simulink model "CF012A_GmStrtStop"  (R2013b)
settings: Solver=FixedStepDiscrete  SolverMode=SingleTasking  StartTime=0.0  StopTime=1  FixedStep=0.002  RelTol=1e-3
values from neighbouring files (symbols this model uses):
  CNV100MICROSECTOMILLISEC_MILLISECPERCNT_F32 = DataDict.Constant    [CF012A_GmStrtStop_DataDict.m]
  DISMOD_CNT_U08 = DataDict.Constant    [CF012A_GmStrtStop_DataDict.m]
  DISMODRATE_ULSPERSEC_F32 = DataDict.Constant    [CF012A_GmStrtStop_DataDict.m]
  FLTMOD_CNT_U08 = DataDict.Constant    [CF012A_GmStrtStop_DataDict.m]
  GmStrtStopEna = DataDict.Calibration    [CF012A_GmStrtStop_DataDict.m]
  GmStrtStopFltRateLim = DataDict.Calibration    [CF012A_GmStrtStop_DataDict.m]
  GmStrtStopMod1ToStopRateLim = DataDict.Calibration    [CF012A_GmStrtStop_DataDict.m]
  GmStrtStopNormRateLim = DataDict.Calibration    [CF012A_GmStrtStop_DataDict.m]
  GmStrtStopNormToMod1RateLim = DataDict.Calibration    [CF012A_GmStrtStop_DataDict.m]
  GmStrtStopStopAndMod2RateLim = DataDict.Calibration    [CF012A_GmStrtStop_DataDict.m]
  GmStrtStopStopMod1Tmr = DataDict.Calibration    [CF012A_GmStrtStop_DataDict.m]
  GmStrtStopStopMod2Tmr = DataDict.Calibration    [CF012A_GmStrtStop_DataDict.m]
  MOD1_CNT_U08 = DataDict.Constant    [CF012A_GmStrtStop_DataDict.m]
  MOD2_CNT_U08 = DataDict.Constant    [CF012A_GmStrtStop_DataDict.m]
  NORMMOD_CNT_U08 = DataDict.Constant    [CF012A_GmStrtStop_DataDict.m]
  STOPMOD_CNT_U08 = DataDict.Constant    [CF012A_GmStrtStop_DataDict.m]
  STRTSTOPRATEHILIM_ULSPERSEC_F32 = DataDict.Constant    [CF012A_GmStrtStop_DataDict.m]
  STRTSTOPRATELOWRLIM_ULSPERSEC_F32 = DataDict.Constant    [CF012A_GmStrtStop_DataDict.m]
  STRTSTOPSCAHILIM_ULS_F32 = DataDict.Constant    [CF012A_GmStrtStop_DataDict.m]
  STRTSTOPSCALOWRLIM_ULS_F32 = DataDict.Constant    [CF012A_GmStrtStop_DataDict.m]
undefined symbols (not defined in the file or in its folder): u2, u3, u4, u5
libraries: FixdToFloat x2, NxtrLim x2, simulink x2
(part 1 of 4)
settings Model: Creator=rzp7hw  LastModifiedBy=sz7vy6
settings SolverCC: AutoInsertRateTranBlk=on  InsertRTBMode=Always
settings DataIOCC: LimitDataPoints=off  SaveFormat=Structure  ReturnWorkspaceOutputs=on
settings OptimizationCC: BlockReduction=off  InlineParams=on  ZeroExternalMemoryAtStartup=off  ZeroInternalMemoryAtStartup=off  OptimizeModelRefInitCode=on  LifeSpan=1
settings DebuggingCC: SignalInfNanChecking=error  SignalRangeChecking=warning  UnderspecifiedInitializationDetection=Simplified  SolverPrmCheckMsg=error  InheritedTsInSrcMsg=error  DiscreteInheritContinuousMsg=error  SingleTaskRateTransMsg=error  TasksWithSamePriorityMsg=error  SigSpecEnsureSampleTimeMsg=error  CheckMatrixSingularityMsg=error  ParameterUnderflowMsg=error  ParameterPrecisionLossMsg=error  ParameterTunabilityLossMsg=error  FixptConstUnderflowMsg=warning  FixptConstOverflowMsg=warning  VectorMatrixConversionMsg=error  SignalLabelMismatchMsg=error  UnconnectedInputMsg=error  UnconnectedOutputMsg=error  UnconnectedLineMsg=error  SFcnCompatibilityMsg=error  UniqueDataStoreMsg=warning  BusObjectLabelMismatch=error  RootOutportRequireBusObject=error  AssertControl=DisableAll  ModelReferenceIOMsg=error  ModelReferenceVersionMismatchMessage=warning  ModelReferenceIOMismatchMessage=error  ModelReferenceCSMismatchMessage=warning  ModelReferenceDataLoggingMessage=error  StateNameClashWarn=warning  StrictBusMsg=ErrorOnBusTreatedAsVector  NonBusSignalsTreatedAsBus=error  SFUnexpectedBacktrackingDiag=error  SFInvalidInputDataAccessInChartInitDiag=error  SFNoUnconditionalDefaultTransitionDiag=error  SFTransitionOutsideNaturalParentDiag=error  SFUnconditionalTransitionShadowingDiag=error  SFUndirectedBroadcastEventsDiag=error
settings ModelReferenceCC: ModelReferenceNumInstancesAllowed=Single
settings RTWCC: SystemTargetFile=autosar.tlc  GenCodeOnly=on  TemplateMakefile=ert_default_tmf  Description=AUTOSAR  GenerateReport=on  ProcessScript=autosar_make_rtw_hook  LaunchReport=on
settings CodeAppCC: GenerateComments=off  IgnoreCustomStorageClasses=off  CustomSymbolStrType=$N$R$M  CustomSymbolStrBlkIO=$N$M  SimulinkBlockComments=off
settings STFCustomTargetCC: ParMdlRefBuildCompliant=on  CompOptLevelCompliant=on  IncludeMdlTerminateFcn=off  CombineOutputUpdateFcns=on  SuppressErrorStatus=on  ERTFirstTimeCompliant=on  ERTCustomFileBanners=on  SupportNonFinite=off  SupportComplex=off  SupportContinuousTime=off  SupportNonInlinedSFcns=off  MATLABClassNameForMDSCustomization=Simulink.SoftwareTarget.ERTCustomization  AutosarCompliant=on  GRTInterface=off  SystemTargetFile=autosar.tlc
settings ERTTargetCC: CodeReplacementLibrary=ANSI_C  ConcurrentExecutionCompliant=off  IncludeMdlTerminateFcn=off  SuppressErrorStatus=on  SupportNonFinite=off  SupportComplex=off  ModelStepFunctionPrototypeControlCompliant=off  CPPClassGenCompliant=off  AutosarCompliant=on  InlinedParameterPlacement=NonHierarchical  ERTCustomFileTemplate=example_file_process.tlc  EnableUserReplacementTypes=on

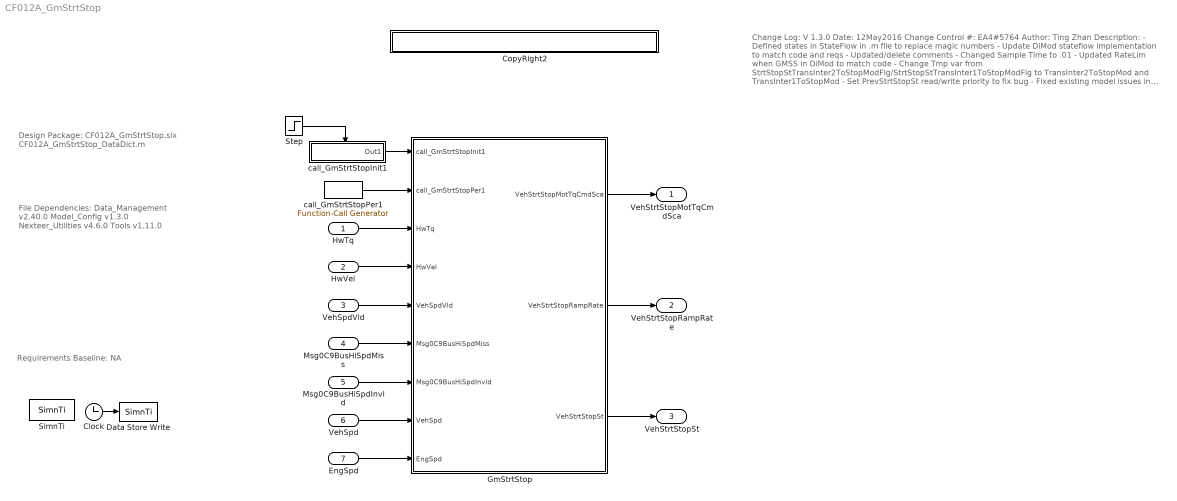
== system CF012A_GmStrtStop ==
  note: File Dependencies:
      |
      | Data_Management v2.40.0
      | Model_Config v1.3.0
      | Nexteer_Utilities v4.6.0
      | Tools v1.11.0
  note: Requirements Baseline: NA
  note: Change Log:
      |
      | V 1.3.0
      | Date: 12May2016
      | Change Control #: EA4#5764
      | Author: Ting Zhan
      |
      | Description:
      | - Defined states in StateFlow in .m file to replace magic numbers
      | - Update DiMod stateflow implementation to match code and reqs
      | - Updated/delete comments
      | - Changed Sample Time to .01
      | - Updated RateLim when GMSS in DiMod to match code
      | - Change Tmp var from StrtStopStTransInter2ToStopModFlg/StrtStopStTransInter1ToStopModFlg
      |  to TransInter2ToStopMod and TransInter1ToStopMod
      | - Set PrevStrtStopSt read/write priority to fix bug
      | - Fixed existing model issues in order to make model run
      |
      | V 1.2.0
      | Date: 08Feb2015
      | Change Control #: EA4#3589
      | Author: Sneha P (KPIT)
      | Description:
      |
      | - Replaced constant “MILLISECTO100MICROSECCNVN_CNT_F32” with
      |  “CNV100MICROSECTOMILLISEC_MILLISECPERCNT_F32“ in .m file
      | - Removed Millisec to 100Microsec coversion logic and implemented
      |   100Microsec(Cnt) to MilliSec conversion logic in model
      | Path:(CF012A_GmStrtStop/GmStrtStop/GmStrtStopPer1/StrtStopSt_Inter2ToStopModFlg/Elpse Ti)
      | and : (CF012A_GmStrtStop/GmStrtStop/GmStrtStopPer1/StrtStopSt_Inter1ToStopModFlg/Elpse Ti)
      | - Changed DocUnit of "GmStrtStopStopMod2Tmr" to "MilliSec" with
      |    respective change in Init, Min, Max values
      |
      |
      | V 1.1.0
      | Date: 29Jan2015
      | Change Control #: EA4#3589
      | Author: Sneha P (KPIT)
      | Description:
      |
      | - Changed maximum range of PIM variables 'PrevStrtStopSt' & 'PrevActSt'
      |   from 4 to 5 as per anomaly EA4#2621
      |
      | - Changed Init value of output signal 'StrtStopSca' from 0 to 1 as per
      |   anomaly CR EA4#3036
      |
      | - Following changes done as per anomaly CR#1886
      |
      |   - In .m file, calibration 'GmStrtStopStopMod1Tmr' changed to 'float32'
      |   - In .m file, PIMS 'Mod1RefTmr' and 'Mod2RefTmr' changed to 'uint32'
      |   - Constant 'TISTEP_MILLISEC_F32' to be removed from .m file.
      |   - Logic related to elapsed timers in state implemented in model
      |
      | - Data type of PIM variables 'Mod1RefTmr' and 'Mod2RefTmr' changed to uint32
      |   as per anomaly CR EA4#2991
      |
      |
      | V 1.0.0
      | Date: 8Jul2015
      | Change Control #: EA4#
      | Author: Qi Wang
      | Description:
      | - Initial Release Based on EA3V 1.0.0
      | CR#1623
  note: Design Package:
      | CF012A_GmStrtStop.slx
      | CF012A_GmStrtStop_DataDict.m
  HwTq : Inport  RequirementInfo={} %GIDa_a4d85b5d_ed9b_4901_a351_104e8322e8d5
  HwVel : Inport  RequirementInfo={} %GIDa_ecdde577_07ed_48f6_83d9_055f4ed5439e  Port=2
  VehSpdVld : Inport  Port=3
  Msg0C9BusHiSpdMiss : Inport  Port=4
  Msg0C9BusHiSpdInvld : Inport  Port=5
  VehSpd : Inport  RequirementInfo={} %GIDa_7789dff7_ea50_483a_835d_9871b9cb485d  Port=6
  EngSpd : Inport  RequirementInfo={} %GIDa_55b73ebd_28f3_4154_b330_73735b6396df  Port=7
  Clock : Clock
  CopyRight2 : Subsystem  Description=|  mask(Copyright Information){none=on}
      | Copyright info block.                                               
      |                                                                     
      | Place copyright information at the top of every subsystem in design.
      mask prompts: none "No parameters"
      mask help: Place copyright information at the top of every subsystem in design.
      mask Display:
      | NxtrConf = 'Nexteer Confidential';
      | 
      | sys = bdroot; %handle for the current model ("system")
      | first = get_param(sys,'Created');
      | if(isempty(first))
      |     first = datestr(now,'yyyy');
      | else
      |     first = first(end-3:end);  %year is last four digits
      | end
      | 
      | last = get_param(sys,'LastModifiedDate');
      | if isempty(last)
      |     last = datestr(now,'yyyy');
      | else
      |     last = last(end-3:end);
      | end
      | 
      | if strcmp(first,last)
      |     fprintf('%s -- Copyright %s Nexteer',NxtrConf,first)
      | else
      |     fprintf('%s -- %s%s- %s Nexteer',NxtrConf,char(169),first,last)
      | end
  Data Store Write : DataStoreWrite  DataStoreName=SimnTi
  GmStrtStop : Subsystem  RequirementInfo={} %GIDa_2223a9a7_07d3_48cf_9066_a6e132ab91db
  SimnTi : DataStoreMemory  DataStoreName=SimnTi
  Step : Step  Time=.002  Before=1  After=0  SampleTime=0
  call_GmStrtStopInit1 : Subsystem  TreatAsAtomicUnit=on
  call_GmStrtStopPer1 : simulink/Ports & Subsystems/Function-Call Generator  RequirementInfo={} %GIDa_054eadac_8b4f_4392_b7a2_0fbd071b25ae  sample_time=.01  numberOfIterations=1
      settings: AttributesFormatString=%<sample_time>
  VehStrtStopMotTqCmdSca : Outport  RequirementInfo={} %GIDa_bfe28696_5cd6_4f13_a500_f4d97106e76f
  VehStrtStopRampRate : Outport  RequirementInfo={} %GIDa_064db67c_6e20_4c88_b4e7_4e0dfc6b8609  Port=2
  VehStrtStopSt : Outport  RequirementInfo={} %GIDa_5adf65af_5735_4113_a387_e1ee48936d3d  Port=3
  wires:
  call_GmStrtStopPer1/1 -> GmStrtStop/2(call_GmStrtStopPer1)
  HwTq/1 -> GmStrtStop/3(HwTq)
  HwVel/1 -> GmStrtStop/4(HwVel)
  VehSpdVld/1 -> GmStrtStop/5(VehSpdVld)
  Msg0C9BusHiSpdMiss/1 -> GmStrtStop/6(Msg0C9BusHiSpdMiss)
  Msg0C9BusHiSpdInvld/1 -> GmStrtStop/7(Msg0C9BusHiSpdInvld)
  VehSpd/1 -> GmStrtStop/8(VehSpd)
  EngSpd/1 -> GmStrtStop/9(EngSpd)
  GmStrtStop/1(VehStrtStopMotTqCmdSca) -> VehStrtStopMotTqCmdSca/1
  GmStrtStop/2(VehStrtStopRampRate) -> VehStrtStopRampRate/1
  GmStrtStop/3(VehStrtStopSt) -> VehStrtStopSt/1
  Step/1 -> call_GmStrtStopInit1/Enable
  call_GmStrtStopInit1/1(Out1) -> GmStrtStop/1(call_GmStrtStopInit1)
  Clock/1 -> Data Store Write/1

== system CF012A_GmStrtStop/CopyRight2 ==

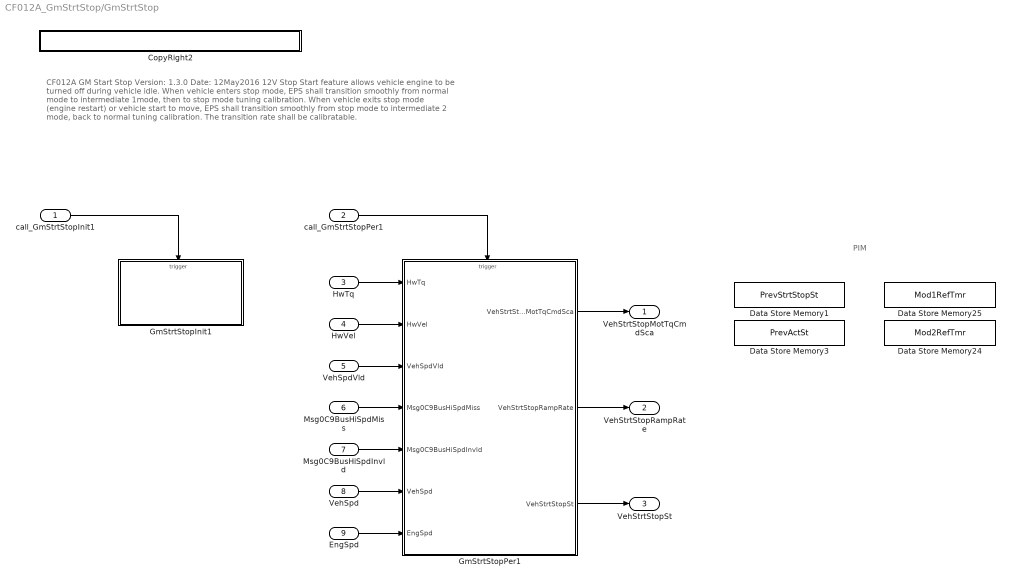
== system CF012A_GmStrtStop/GmStrtStop ==
  note: PIM
  note: CF012A GM Start Stop
      | Version: 1.3.0      Date: 12May2016
      |
      | 12V Stop Start feature allows vehicle engine to be turned off during vehicle idle. When vehicle enters stop mode, EPS shall transition smoothly from
      | normal mode to intermediate 1mode, then to stop mode tuning calibration.  When vehicle exits stop mode (engine restart) or vehicle start to move, EPS shall
      | transition smoothly from stop mode to intermediate 2 mode, back to normal tuning calibration.  The transition rate shall be calibratable.
  call_GmStrtStopInit1 : Inport  RequirementInfo={} %GIDa_e66133ce_4d9a_4583_9cdf_9b3fe85f0c43
  call_GmStrtStopPer1 : Inport  RequirementInfo={} %GIDa_29356ae4_ffe9_446f_a246_ff587b699871  Port=2
  HwTq : Inport  RequirementInfo="{'linktype_rmi_doors' '0000c6e0 (/GM T1XX/SubSystem Specifications/Customer Functions/CF012 12V Start Stop)' '#9' 'true' 'REQ:  9' '' } %GIDa_b59c9030_1f31_468f_8592_3e6a0470c9b8"  Port=3
  HwVel : Inport  RequirementInfo="{'linktype_rmi_doors' '0000c6e0 (/GM T1XX/SubSystem Specifications/Customer Functions/CF012 12V Start Stop)' '#32' 'true' 'REQ:  32' '' } %GIDa_d97376d2_3983_4ccc_a2b9_13e32f4f2e19"  Port=4
  VehSpdVld : Inport  RequirementInfo="{'linktype_rmi_doors' '0000c6e0 (/GM T1XX/SubSystem Specifications/Customer Functions/CF012 12V Start Stop)' '#33' 'true' 'REQ:  33' '' } %GIDa_855152bf_675c_4d82_87df_76d2e9253c11"  Port=5
  Msg0C9BusHiSpdMiss : Inport  RequirementInfo="{'linktype_rmi_doors' '0000c6e0 (/GM T1XX/SubSystem Specifications/Customer Functions/CF012 12V Start Stop)' '#73' 'true' 'REQ:  73' '' } %GIDa_4764eb12_da95_4964_a18b_bc9ea30562ea"  Port=6
  Msg0C9BusHiSpdInvld : Inport  RequirementInfo="{'linktype_rmi_doors' '0000c6e0 (/GM T1XX/SubSystem Specifications/Customer Functions/CF012 12V Start Stop)' '#221' 'true' 'REQ:  221' '' } %GIDa_0435394c_4b65_4e7a_927b_eb164670af9f"  Port=7
  VehSpd : Inport  RequirementInfo="{'linktype_rmi_doors' '0000c6e0 (/GM T1XX/SubSystem Specifications/Customer Functions/CF012 12V Start Stop)' '#36' 'true' 'REQ:  36' '' } %GIDa_26fe1dc3_440c_4c24_809e_674d3c570084"  Port=8
  EngSpd : Inport  RequirementInfo="{'linktype_rmi_doors' '0000c6e0 (/GM T1XX/SubSystem Specifications/Customer Functions/CF012 12V Start Stop)' '#37' 'true' 'REQ:  37' '' } %GIDa_1a15c7f1_c702_477b_b228_a391a493889d"  Port=9
  CopyRight2 : Subsystem  Description=|  mask(Copyright Information){none=on}
      | Copyright info block.                                               
      |                                                                     
      | Place copyright information at the top of every subsystem in design.
      mask prompts: none "No parameters"
      mask help: Place copyright information at the top of every subsystem in design.
      mask Display:
      | NxtrConf = 'Nexteer Confidential';
      | 
      | sys = bdroot; %handle for the current model ("system")
      | first = get_param(sys,'Created');
      | if(isempty(first))
      |     first = datestr(now,'yyyy');
      | else
      |     first = first(end-3:end);  %year is last four digits
      | end
      | 
      | last = get_param(sys,'LastModifiedDate');
      | if isempty(last)
      |     last = datestr(now,'yyyy');
      | else
      |     last = last(end-3:end);
      | end
      | 
      | if strcmp(first,last)
      |     fprintf('%s -- Copyright %s Nexteer',NxtrConf,first)
      | else
      |     fprintf('%s -- %s%s- %s Nexteer',NxtrConf,char(169),first,last)
      | end
  Data Store Memory1 : DataStoreMemory  DataStoreName=PrevStrtStopSt  StateMustResolveToSignalObject=on
  Data Store Memory24 : DataStoreMemory  DataStoreName=Mod2RefTmr  StateMustResolveToSignalObject=on
  Data Store Memory25 : DataStoreMemory  DataStoreName=Mod1RefTmr  StateMustResolveToSignalObject=on
  Data Store Memory3 : DataStoreMemory  DataStoreName=PrevActSt  StateMustResolveToSignalObject=on
  GmStrtStopInit1 : Subsystem
  GmStrtStopPer1 : Subsystem
  VehStrtStopMotTqCmdSca : Outport  RequirementInfo="{'linktype_rmi_doors' '0000c6e0 (/GM T1XX/SubSystem Specifications/Customer Functions/CF012 12V Start Stop)' '#11' 'true' 'REQ:  11' '' } %GIDa_548d980c_3c7b_491e_a0fa_0c64e6562fc0"
  VehStrtStopRampRate : Outport  RequirementInfo="{'linktype_rmi_doors' '0000c6e0 (/GM T1XX/SubSystem Specifications/Customer Functions/CF012 12V Start Stop)' '#40' 'true' 'REQ:  40' '' } %GIDa_43ddaf5d_aaf1_4964_b6d5_b32b85f57a27"  Port=2
  VehStrtStopSt : Outport  RequirementInfo="{'linktype_rmi_doors' '0000c6e0 (/GM T1XX/SubSystem Specifications/Customer Functions/CF012 12V Start Stop)' '#216' 'true' 'REQ:  216' '' } %GIDa_fd34a469_cf67_4bd9_a2b8_b0cdcd42aa93"  Port=3
  wires:
  HwTq/1 -> GmStrtStopPer1/1(HwTq)
  HwVel/1 -> GmStrtStopPer1/2(HwVel)
  VehSpd/1 -> GmStrtStopPer1/6(VehSpd)
  EngSpd/1 -> GmStrtStopPer1/7(EngSpd)
  GmStrtStopPer1/1(VehStrtStopMotTqCmdSca) -> VehStrtStopMotTqCmdSca/1
  GmStrtStopPer1/2(VehStrtStopRampRate) -> VehStrtStopRampRate/1
  call_GmStrtStopPer1/1 -> GmStrtStopPer1/Trigger
  GmStrtStopPer1/3(VehStrtStopSt) -> VehStrtStopSt/1
  Msg0C9BusHiSpdInvld/1 -> GmStrtStopPer1/5(Msg0C9BusHiSpdInvld)
  Msg0C9BusHiSpdMiss/1 -> GmStrtStopPer1/4(Msg0C9BusHiSpdMiss)
  VehSpdVld/1 -> GmStrtStopPer1/3(VehSpdVld)
  call_GmStrtStopInit1/1 -> GmStrtStopInit1/Trigger

== system CF012A_GmStrtStop/call_GmStrtStopInit1 ==
  Enable : EnablePort
  CopyRight2 : Subsystem  Description=|  mask(Copyright Information){none=on}
      | Copyright info block.                                               
      |                                                                     
      | Place copyright information at the top of every subsystem in design.
      mask prompts: none "No parameters"
      mask help: Place copyright information at the top of every subsystem in design.
      mask Display:
      | NxtrConf = 'Nexteer Confidential';
      | 
      | sys = bdroot; %handle for the current model ("system")
      | first = get_param(sys,'Created');
      | if(isempty(first))
      |     first = datestr(now,'yyyy');
      | else
      |     first = first(end-3:end);  %year is last four digits
      | end
      | 
      | last = get_param(sys,'LastModifiedDate');
      | if isempty(last)
      |     last = datestr(now,'yyyy');
      | else
      |     last = last(end-3:end);
      | end
      | 
      | if strcmp(first,last)
      |     fprintf('%s -- Copyright %s Nexteer',NxtrConf,first)
      | else
      |     fprintf('%s -- %s%s- %s Nexteer',NxtrConf,char(169),first,last)
      | end
  Function-Call Generator : simulink/Ports & Subsystems/Function-Call Generator  sample_time=.01  numberOfIterations=1
  Out1 : Outport
  wires:
  Function-Call Generator/1 -> Out1/1

== system CF012A_GmStrtStop/GmStrtStop/CopyRight2 ==

== system CF012A_GmStrtStop/GmStrtStop/GmStrtStopInit1 ==
  function : TriggerPort  TriggerType=function-call
  CopyRight2 : Subsystem  Description=|  mask(Copyright Information){none=on}
      | Copyright info block.                                               
      |                                                                     
      | Place copyright information at the top of every subsystem in design.
      mask prompts: none "No parameters"
      mask help: Place copyright information at the top of every subsystem in design.
      mask Display:
      | NxtrConf = 'Nexteer Confidential';
      | 
      | sys = bdroot; %handle for the current model ("system")
      | first = get_param(sys,'Created');
      | if(isempty(first))
      |     first = datestr(now,'yyyy');
      | else
      |     first = first(end-3:end);  %year is last four digits
      | end
      | 
      | last = get_param(sys,'LastModifiedDate');
      | if isempty(last)
      |     last = datestr(now,'yyyy');
      | else
      |     last = last(end-3:end);
      | end
      | 
      | if strcmp(first,last)
      |     fprintf('%s -- Copyright %s Nexteer',NxtrConf,first)
      | else
      |     fprintf('%s -- %s%s- %s Nexteer',NxtrConf,char(169),first,last)
      | end
  Data Store Write4 : DataStoreWrite  RequirementInfo="{'linktype_rmi_doors' '0000c6e0 (/GM T1XX/SubSystem Specifications/Customer Functions/CF012 12V Start Stop)' '#161' 'true' 'REQ:  161' '' } %GIDa_5ca1f0f5_5840_49db_9093_aa24770101e9"  DataStoreName=Mod2RefTmr
  Data Store Write5 : DataStoreWrite  RequirementInfo="{'linktype_rmi_doors' '0000c6e0 (/GM T1XX/SubSystem Specifications/Customer Functions/CF012 12V Start Stop)' '#149' 'true' 'REQ:  149' '' } %GIDa_d8f43907_f50d_4586_b279_7eacc1f075da"  DataStoreName=Mod1RefTmr
  GetRefTmr100MicroSec32bit : Subsystem  RequirementInfo="{'linktype_rmi_doors' '0000c6e0 (/GM T1XX/SubSystem Specifications/Customer Functions/CF012 12V Start Stop)' '#161' 'true' 'REQ:  161' '' ; 'linktype_rmi_doors' '0000c6e0 (/GM T1XX/SubSystem Specifications/Customer Functions/CF012 12V Start Stop)' '#149' 'true' 'REQ:  149' '' } %GIDa_033bf37f_1dc6_42f0_a9e6_3056b3737b66"
  wires:
  GetRefTmr100MicroSec32bit/1(RefTmr) -> Data Store Write4/1, Data Store Write5/1

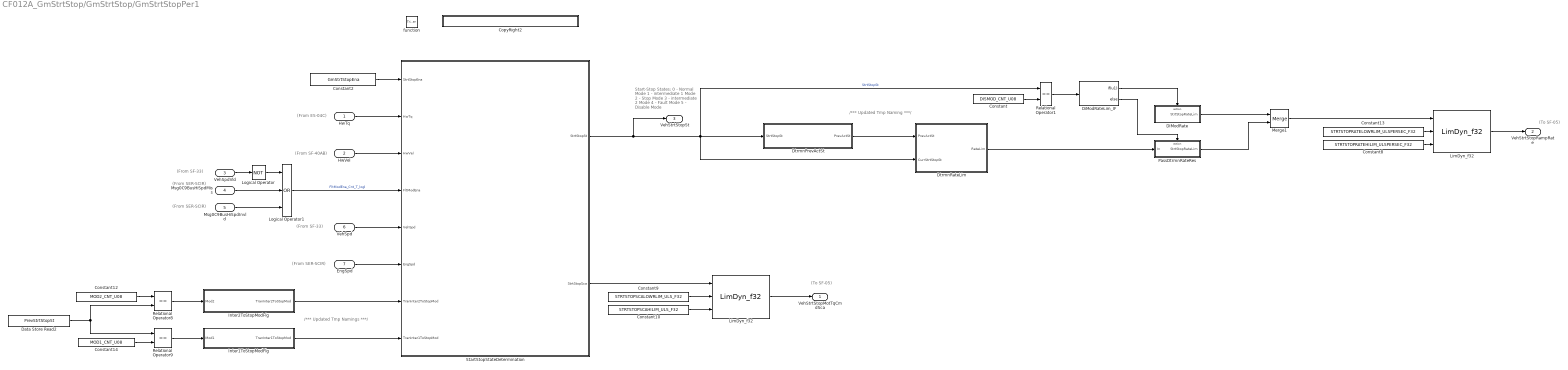
== system CF012A_GmStrtStop/GmStrtStop/GmStrtStopPer1 ==
  note: (From SER-SCIR)
  note: (From SF-33)
  note: (From SF-33)
  note: (From ES-04C)
  note: (From SF-40AB)
  note: Start-Stop States:
      |     0 - Normal Mode
      |     1 - intermediate 1 Mode
      |     2 - Stop Mode
      |     3 - intermediate 2 Mode
      |     4 - Fault Mode
      |     5 - Disable Mode
  note: (To SF-05)
  note: (To SF-05)
  note: (From SER-SCIR)
  note: (From SER-SCIR)
  note: /*** Updated Tmp Naming ***/
  note: /*** Updated Tmp Namings ***/
  HwTq : Inport  RequirementInfo="{'linktype_rmi_doors' '0000c6e0 (/GM T1XX/SubSystem Specifications/Customer Functions/CF012 12V Start Stop)' '#9' 'true' 'REQ:  9' '' } %GIDa_42b69aa0_42a4_4740_8c59_976a11e7f2ed"
  HwVel : Inport  RequirementInfo="{'linktype_rmi_doors' '0000c6e0 (/GM T1XX/SubSystem Specifications/Customer Functions/CF012 12V Start Stop)' '#32' 'true' 'REQ:  32' '' } %GIDa_ce32f278_8b5d_4046_b147_1f30eda0ac5e"  Port=2
  VehSpdVld : Inport  RequirementInfo="{'linktype_rmi_doors' '0000c6e0 (/GM T1XX/SubSystem Specifications/Customer Functions/CF012 12V Start Stop)' '#33' 'true' 'REQ:  33' '' } %GIDa_5065ff7a_d581_4098_bd8a_dd99a06fb2d8"  Port=3
  Msg0C9BusHiSpdMiss : Inport  RequirementInfo="{'linktype_rmi_doors' '0000c6e0 (/GM T1XX/SubSystem Specifications/Customer Functions/CF012 12V Start Stop)' '#73' 'true' 'REQ:  73' '' } %GIDa_81f8689f_bedf_48cc_9965_5d5e08e37da1"  Port=4
  Msg0C9BusHiSpdInvld : Inport  RequirementInfo="{'linktype_rmi_doors' '0000c6e0 (/GM T1XX/SubSystem Specifications/Customer Functions/CF012 12V Start Stop)' '#221' 'true' 'REQ:  221' '' } %GIDa_2c4353c3_7199_496f_b5e4_ca48d4fdc361"  Port=5
  VehSpd : Inport  RequirementInfo="{'linktype_rmi_doors' '0000c6e0 (/GM T1XX/SubSystem Specifications/Customer Functions/CF012 12V Start Stop)' '#36' 'true' 'REQ:  36' '' } %GIDa_778ed2e2_bf34_46d0_bd92_dde0215ed3d0"  Port=6
  EngSpd : Inport  RequirementInfo="{'linktype_rmi_doors' '0000c6e0 (/GM T1XX/SubSystem Specifications/Customer Functions/CF012 12V Start Stop)' '#37' 'true' 'REQ:  37' '' } %GIDa_ceeb79ba_05d2_485d_8198_e45df6d9a78c"  Port=7
  function : TriggerPort  TriggerType=function-call
  Constant : Constant  RequirementInfo="{'linktype_rmi_doors' '0000c6e0 (/GM T1XX/SubSystem Specifications/Customer Functions/CF012 12V Start Stop)' '#224' 'true' 'REQ:  224' '' } %GIDa_561b1e7e_3960_4a83_833c_80ef798b62ac"  Value=DISMOD_CNT_U08
  Constant10 : Constant  RequirementInfo="{'linktype_rmi_doors' '0000c6e0 (/GM T1XX/SubSystem Specifications/Customer Functions/CF012 12V Start Stop)' '#11' 'true' 'REQ:  11' '' } %GIDa_0c487a41_a1a4_450c_934d_c18e6ddbeebb"  Value=STRTSTOPSCAHILIM_ULS_F32
  Constant12 : Constant  RequirementInfo="{'linktype_rmi_doors' '0000c6e0 (/GM T1XX/SubSystem Specifications/Customer Functions/CF012 12V Start Stop)' '#161' 'true' 'REQ:  161' '' } %GIDa_bd66a335_3060_4277_b6ba_17e2ef32d7e1"  Value=MOD2_CNT_U08
  Constant13 : Constant  RequirementInfo="{'linktype_rmi_doors' '0000c6e0 (/GM T1XX/SubSystem Specifications/Customer Functions/CF012 12V Start Stop)' '#40' 'true' 'REQ:  40' '' } %GIDa_7a48ffb4_78e6_42f2_aec5_f8db377a48d6"  Value=STRTSTOPRATELOWRLIM_ULSPERSEC_F32
  Constant14 : Constant  RequirementInfo="{'linktype_rmi_doors' '0000c6e0 (/GM T1XX/SubSystem Specifications/Customer Functions/CF012 12V Start Stop)' '#149' 'true' 'REQ:  149' '' } %GIDa_d624ad54_41a1_4556_8a85_b9999226efec"  Value=MOD1_CNT_U08
  Constant2 : Constant  RequirementInfo="{'linktype_rmi_doors' '0000c6e0 (/GM T1XX/SubSystem Specifications/Customer Functions/CF012 12V Start Stop)' '#167' 'true' 'REQ:  167' '' ; 'linktype_rmi_doors' '0000c6e0 (/GM T1XX/SubSystem Specifications/Customer Functions/CF012 12V Start Stop)' '#225' 'true' 'REQ:  225' '' } %GIDa_4a6d5448_9282_48ab_99f6_9d1d9d9c576e"  Value=GmStrtStopEna  OutDataTypeStr=single
  Constant8 : Constant  RequirementInfo="{'linktype_rmi_doors' '0000c6e0 (/GM T1XX/SubSystem Specifications/Customer Functions/CF012 12V Start Stop)' '#40' 'true' 'REQ:  40' '' } %GIDa_a36f5600_300f_402a_9cfb_cda0992e5733"  Value=STRTSTOPRATEHILIM_ULSPERSEC_F32
  Constant9 : Constant  RequirementInfo="{'linktype_rmi_doors' '0000c6e0 (/GM T1XX/SubSystem Specifications/Customer Functions/CF012 12V Start Stop)' '#11' 'true' 'REQ:  11' '' } %GIDa_09a6d7e0_4b74_46ca_8329_69c0f542f506"  Value=STRTSTOPSCALOWRLIM_ULS_F32
  CopyRight2 : Subsystem  Description=|  mask(Copyright Information){none=on}
      | Copyright info block.                                               
      |                                                                     
      | Place copyright information at the top of every subsystem in design.
      mask prompts: none "No parameters"
      mask help: Place copyright information at the top of every subsystem in design.
      mask Display:
      | NxtrConf = 'Nexteer Confidential';
      | 
      | sys = bdroot; %handle for the current model ("system")
      | first = get_param(sys,'Created');
      | if(isempty(first))
      |     first = datestr(now,'yyyy');
      | else
      |     first = first(end-3:end);  %year is last four digits
      | end
      | 
      | last = get_param(sys,'LastModifiedDate');
      | if isempty(last)
      |     last = datestr(now,'yyyy');
      | else
      |     last = last(end-3:end);
      | end
      | 
      | if strcmp(first,last)
      |     fprintf('%s -- Copyright %s Nexteer',NxtrConf,first)
      | else
      |     fprintf('%s -- %s%s- %s Nexteer',NxtrConf,char(169),first,last)
      | end
  DIModRate : Subsystem  RequirementInfo="{'linktype_rmi_doors' '0000c6e0 (/GM T1XX/SubSystem Specifications/Customer Functions/CF012 12V Start Stop)' '#224' 'true' 'REQ:  224' '' } %GIDa_cf64ce6a_5fba_49e3_8042_142212826b91"  TreatAsAtomicUnit=on
  Data Store Read2 : DataStoreRead  RequirementInfo="{'linktype_rmi_doors' '0000c6e0 (/GM T1XX/SubSystem Specifications/Customer Functions/CF012 12V Start Stop)' '#149' 'true' 'REQ:  149' '' ; 'linktype_rmi_doors' '0000c6e0 (/GM T1XX/SubSystem Specifications/Customer Functions/CF012 12V Start Stop)' '#161' 'true' 'REQ:  161' '' } %GIDa_8d9c1ce9_7c89_423f_9be9_4e5c944f3999"  DataStoreName=PrevStrtStopSt
  DiModRateLim_IF : If  RequirementInfo="{'linktype_rmi_doors' '0000c6e0 (/GM T1XX/SubSystem Specifications/Customer Functions/CF012 12V Start Stop)' '#224' 'true' 'REQ:  224' '' } %GIDa_038e327d_895d_4c44_8a2d_683ea8b3fc41"  IfExpression=u1
  DtrmnPrevActSt : Subsystem  RequirementInfo="{'linktype_rmi_doors' '0000c6e0 (/GM T1XX/SubSystem Specifications/Customer Functions/CF012 12V Start Stop)' '#188' 'true' 'REQ:  188' '' } %GIDa_38faffb5_a6c9_485e_beed_5aff9cc6285a"
  DtrmnRateLim : Subsystem  RequirementInfo="{'linktype_rmi_doors' '0000c6e0 (/GM T1XX/SubSystem Specifications/Customer Functions/CF012 12V Start Stop)' '#86' 'true' 'REQ:  86' '' ; 'linktype_rmi_doors' '0000c6e0 (/GM T1XX/SubSystem Specifications/Customer Functions/CF012 12V Start Stop)' '#86' 'true' 'REQ:  86' '' ; 'linktype_rmi_doors' '0000c6e0 (/GM T1XX/SubSystem Specifications/Customer Functions/CF012 12V Start Stop)' '#86' 'true' 'REQ:  86' '' ; 'linktype_rmi_doors' '0000c6e0 (/GM T1XX/SubSystem Specifications/Customer Functions/CF012 12V Start Stop)' '#86' 'true' 'REQ:  86' '' ; 'linktype_rmi_doors' '0000c6e0 (/GM T1XX/SubSystem Specifications/Customer Functions/CF012 12V Start Stop)' '#86' 'true' 'REQ:  86' '' ; 'linktype_rmi_doors' '0000c6e0 (/GM T1XX/SubSystem Specifications/Customer Functions/CF012 12V Start Stop)' '#86' 'true' 'REQ:  86' '' ; 'linktype_rmi_doors' '0000c6e0 (/GM T1XX/SubSystem Specifications/Customer Functions/CF012 12V Start Stop)' '#86' 'true' 'REQ:  86' '' ; 'linktype_rmi_doors' '0000c6e0 (/GM T1XX/SubSystem Specifications/Customer Functions/CF012 12V Start Stop)' '#86' 'true' 'REQ:  86' '' } %GIDa_299b1b09_a509_4cb4_84f5_ba180b901640"
  Inter1ToStopModFlg : Subsystem  RequirementInfo="{'linktype_rmi_doors' '0000c6e0 (/GM T1XX/SubSystem Specifications/Customer Functions/CF012 12V Start Stop)' '#149' 'true' 'REQ:  149' '' } %GIDa_f6a3c2ac_6653_4871_9b62_0dad353837e0"
  Inter2ToStopModFlg : Subsystem  RequirementInfo="{'linktype_rmi_doors' '0000c6e0 (/GM T1XX/SubSystem Specifications/Customer Functions/CF012 12V Start Stop)' '#161' 'true' 'REQ:  161' '' } %GIDa_237f332d_7f17_42d1_8ac2_b1f2b09eedb1"
  LimDyn_f32 : NxtrLim/LimDyn_f32  RequirementInfo="{'linktype_rmi_doors' '0000c6e0 (/GM T1XX/SubSystem Specifications/Customer Functions/CF012 12V Start Stop)' '#40' 'true' 'REQ:  40' '' } %GIDa_8dd4f5c4_8b44_41f4_a726_2d8ed3933d71"
  "LimDyn_f32 " : NxtrLim/LimDyn_f32  RequirementInfo="{'linktype_rmi_doors' '0000c6e0 (/GM T1XX/SubSystem Specifications/Customer Functions/CF012 12V Start Stop)' '#11' 'true' 'REQ:  11' '' } %GIDa_7f5cde65_aec4_4b2d_989f_08b7e75f57e7"
  Logical Operator : Logic  RequirementInfo="{'linktype_rmi_doors' '0000c6e0 (/GM T1XX/SubSystem Specifications/Customer Functions/CF012 12V Start Stop)' '#62' 'true' 'REQ:  62' '' } %GIDa_656b04b2_cd99_48f1_ac88_88cf48a7ecb0"  Operator=NOT  AllPortsSameDT=off  OutDataTypeStr=boolean
  Logical Operator1 : Logic  RequirementInfo="{'linktype_rmi_doors' '0000c6e0 (/GM T1XX/SubSystem Specifications/Customer Functions/CF012 12V Start Stop)' '#62' 'true' 'REQ:  62' '' } %GIDa_76727bc4_1e34_4aba_9373_5b27799bfd27"  Operator=OR  Inputs=3  AllPortsSameDT=off  OutDataTypeStr=boolean
  Merge1 : Merge  RequirementInfo="{'linktype_rmi_doors' '0000c6e0 (/GM T1XX/SubSystem Specifications/Customer Functions/CF012 12V Start Stop)' '#224' 'true' 'REQ:  224' '' } %GIDa_d024fa85_1cfa_401c_a369_23d7beb805e7"
  PassDtrmnRateRes : Subsystem  RequirementInfo="{'linktype_rmi_doors' '0000c6e0 (/GM T1XX/SubSystem Specifications/Customer Functions/CF012 12V Start Stop)' '#224' 'true' 'REQ:  224' '' } %GIDa_3f3bc633_468d_4c4a_b40c_e9cb87a46491"  TreatAsAtomicUnit=on
  Relational Operator1 : RelationalOperator  RequirementInfo="{'linktype_rmi_doors' '0000c6e0 (/GM T1XX/SubSystem Specifications/Customer Functions/CF012 12V Start Stop)' '#224' 'true' 'REQ:  224' '' } %GIDa_4e8ea01d_c3d6_4af6_979b_c7f1ad0648af"  Operator===  OutDataTypeStr=boolean
  Relational Operator8 : RelationalOperator  RequirementInfo="{'linktype_rmi_doors' '0000c6e0 (/GM T1XX/SubSystem Specifications/Customer Functions/CF012 12V Start Stop)' '#161' 'true' 'REQ:  161' '' } %GIDa_33121b5f_7920_406b_86ac_c7c8173ab72f"  Operator===  OutDataTypeStr=boolean
  Relational Operator9 : RelationalOperator  RequirementInfo="{'linktype_rmi_doors' '0000c6e0 (/GM T1XX/SubSystem Specifications/Customer Functions/CF012 12V Start Stop)' '#149' 'true' 'REQ:  149' '' } %GIDa_4c13c417_adfb_409e_9fd6_df832113dce8"  Operator===  OutDataTypeStr=boolean
  StartStopStateDetermination : Stateflow chart  RequirementInfo="{'linktype_rmi_doors' '0000c6e0 (/GM T1XX/SubSystem Specifications/Customer Functions/CF012 12V Start Stop)' '#86' 'true' 'REQ:  86' '' ; 'linktype_rmi_doors' '0000c6e0 (/GM T1XX/SubSystem Specifications/Customer Functions/CF012 12V Start Stop)' '#166' 'true' 'REQ:  166' '' } %GIDa_c43b243b_0ee6_40fb_9826_be8530fa02b0"  TreatAsAtomicUnit=on  VariantControl=Variant1
  VehStrtStopMotTqCmdSca : Outport  RequirementInfo="{'linktype_rmi_doors' '0000c6e0 (/GM T1XX/SubSystem Specifications/Customer Functions/CF012 12V Start Stop)' '#11' 'true' 'REQ:  11' '' } %GIDa_cf5c80f6_4e22_46d3_8a7e_cf1a6ce51e5a"
  VehStrtStopRampRate : Outport  RequirementInfo="{'linktype_rmi_doors' '0000c6e0 (/GM T1XX/SubSystem Specifications/Customer Functions/CF012 12V Start Stop)' '#40' 'true' 'REQ:  40' '' } %GIDa_bd18f9ff_e11a_445b_ba9a_868b7e7cdcb3"  Port=2
  VehStrtStopSt : Outport  RequirementInfo="{'linktype_rmi_doors' '0000c6e0 (/GM T1XX/SubSystem Specifications/Customer Functions/CF012 12V Start Stop)' '#216' 'true' 'REQ:  216' '' } %GIDa_3f167dff_2f2a_4c61_8d63_f420465aae9f"  Port=3
  wires:
  HwVel/1 -> StartStopStateDetermination/3(HwVel)
  Logical Operator1/1 -> StartStopStateDetermination/4(FltModEna)  "FltModEna_Cnt_T_logl"
  EngSpd/1 -> StartStopStateDetermination/6(EngSpd)
  VehSpd/1 -> StartStopStateDetermination/5(VehSpd)
  HwTq/1 -> StartStopStateDetermination/2(HwTq)
  Constant2/1 -> StartStopStateDetermination/1(StrtStopEna)
  "LimDyn_f32 "/1 -> VehStrtStopMotTqCmdSca/1
  VehSpdVld/1 -> Logical Operator/1
  Logical Operator/1 -> Logical Operator1/1
  Msg0C9BusHiSpdMiss/1 -> Logical Operator1/2
  Msg0C9BusHiSpdInvld/1 -> Logical Operator1/3
  Constant/1 -> Relational Operator1/2
  Relational Operator1/1 -> DiModRateLim_IF/1
  DiModRateLim_IF/1 -> DIModRate/Action
  DiModRateLim_IF/2 -> PassDtrmnRateRes/Action
  PassDtrmnRateRes/1(StrtStopRateLim) -> Merge1/2
  DIModRate/1(StrtStopRateLim) -> Merge1/1
  StartStopStateDetermination/1(StrtStopSt) -> Relational Operator1/1, DtrmnPrevActSt/1(StrtStopSt), DtrmnRateLim/2(CurrStrtStopSt), VehStrtStopSt/1  "StrtStopSt"
  Constant8/1 -> LimDyn_f32/3
  Constant13/1 -> LimDyn_f32/2
  Constant12/1 -> Relational Operator8/1
  Data Store Read2/1 -> Relational Operator8/2, Relational Operator9/1
  Constant14/1 -> Relational Operator9/2
  Relational Operator8/1 -> Inter2ToStopModFlg/1(Mod2)
  Inter2ToStopModFlg/1(TranInter2ToStopMod) -> StartStopStateDetermination/7(TranInter2ToStopMod)
  Inter1ToStopModFlg/1(TranInter1ToStopMod) -> StartStopStateDetermination/8(TranInter1ToStopMod)
  Relational Operator9/1 -> Inter1ToStopModFlg/1(Mod1)
  Constant9/1 -> "LimDyn_f32 "/2
  Constant10/1 -> "LimDyn_f32 "/3
  StartStopStateDetermination/2(StrtStopSca) -> "LimDyn_f32 "/1
  Merge1/1 -> LimDyn_f32/1
  DtrmnRateLim/1(RateLim) -> PassDtrmnRateRes/1(In)
  DtrmnPrevActSt/1(PrevActSt) -> DtrmnRateLim/1(PrevActSt)
  LimDyn_f32/1 -> VehStrtStopRampRate/1

== system CF012A_GmStrtStop/call_GmStrtStopInit1/CopyRight2 ==

== system CF012A_GmStrtStop/GmStrtStop/GmStrtStopInit1/CopyRight2 ==

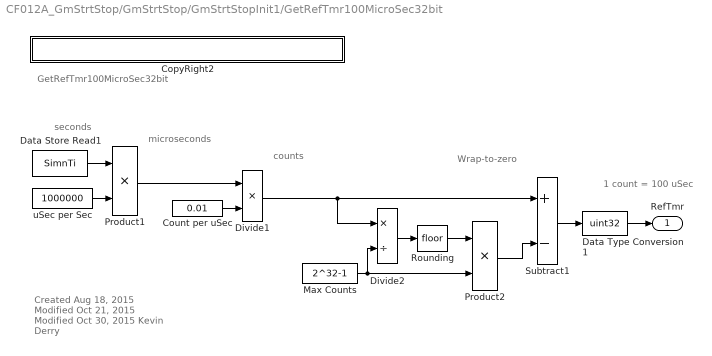
== system CF012A_GmStrtStop/GmStrtStop/GmStrtStopInit1/GetRefTmr100MicroSec32bit ==
  note: Created Aug 18, 2015
      | Modified Oct 21, 2015
      | Modified Oct 30, 2015
      | Kevin Derry
  note: GetRefTmr100MicroSec32bit
  note: Wrap-to-zero
  note: counts
  note: microseconds
  note: seconds
  note: 1 count = 100 uSec
  CopyRight2 : Subsystem  Description=|  mask(Copyright Information){none=on}
      | Copyright info block.                                               
      |                                                                     
      | Place copyright information at the top of every subsystem in design.
      mask prompts: none "No parameters"
      mask help: Place copyright information at the top of every subsystem in design.
      mask Display:
      | NxtrConf = 'Nexteer Confidential';
      | 
      | sys = bdroot; %handle for the current model ("system")
      | first = get_param(sys,'Created');
      | if(isempty(first))
      |     first = datestr(now,'yyyy');
      | else
      |     first = first(end-3:end);  %year is last four digits
      | end
      | 
      | last = get_param(sys,'LastModifiedDate');
      | if isempty(last)
      |     last = datestr(now,'yyyy');
      | else
      |     last = last(end-3:end);
      | end
      | 
      | if strcmp(first,last)
      |     fprintf('%s -- Copyright %s Nexteer',NxtrConf,first)
      | else
      |     fprintf('%s -- %s%s- %s Nexteer',NxtrConf,char(169),first,last)
      | end
  Count per uSec : Constant  Value=0.01
  Data Store Read1 : DataStoreRead  DataStoreName=SimnTi
  Data Type Conversion1 : DataTypeConversion  OutDataTypeStr=uint32
  Divide1 : Product  Inputs=**
  Divide2 : Product  Inputs=*/
  Max Counts : Constant  Value=2^32-1
  Product1 : Product
  Product2 : Product
  Rounding : Rounding
  Subtract1 : Sum  Inputs=+-
  uSec per Sec : Constant  Value=1000000
  RefTmr : Outport
  wires:
  Data Store Read1/1 -> Product1/1
  Data Type Conversion1/1 -> RefTmr/1
  uSec per Sec/1 -> Product1/2
  Count per uSec/1 -> Divide1/2
  Product1/1 -> Divide1/1
  Divide1/1 -> Subtract1/1, Divide2/1
  Max Counts/1 -> Product2/2, Divide2/2
  Divide2/1 -> Rounding/1
  Rounding/1 -> Product2/1
  Subtract1/1 -> Data Type Conversion1/1
  Product2/1 -> Subtract1/2

== system CF012A_GmStrtStop/GmStrtStop/GmStrtStopPer1/CopyRight2 ==

== system CF012A_GmStrtStop/GmStrtStop/GmStrtStopPer1/DIModRate ==
  Action Port : ActionPort  ActionType=then
  Constant1 : Constant  Value=DISMODRATE_ULSPERSEC_F32
  CopyRight2 : Subsystem  Description=|  mask(Copyright Information){none=on}
      | Copyright info block.                                               
      |                                                                     
      | Place copyright information at the top of every subsystem in design.
      mask prompts: none "No parameters"
      mask help: Place copyright information at the top of every subsystem in design.
      mask Display:
      | NxtrConf = 'Nexteer Confidential';
      | 
      | sys = bdroot; %handle for the current model ("system")
      | first = get_param(sys,'Created');
      | if(isempty(first))
      |     first = datestr(now,'yyyy');
      | else
      |     first = first(end-3:end);  %year is last four digits
      | end
      | 
      | last = get_param(sys,'LastModifiedDate');
      | if isempty(last)
      |     last = datestr(now,'yyyy');
      | else
      |     last = last(end-3:end);
      | end
      | 
      | if strcmp(first,last)
      |     fprintf('%s -- Copyright %s Nexteer',NxtrConf,first)
      | else
      |     fprintf('%s -- %s%s- %s Nexteer',NxtrConf,char(169),first,last)
      | end
  StrtStopRateLim : Outport
  wires:
  Constant1/1 -> StrtStopRateLim/1
